simulink subsystem "subsistema_magnetico_estator"  (R2023b)
settings: Solver=VariableStepAuto  StartTime=0.0  StopTime=10.0  RelTol=1e-3
values from neighbouring files (symbols this model uses):
  L_d = 6.6    [main.m]    (also in parametros.m = 0.0066)
  L_q = 5.8e-3    (= 0.0058)    [diagrama_polos_y_ceros_LTI.m]    (also in main.m = 5.8; parametros.m; variacion_de_parametros.m)
  lambda_m = 0.016    [main.m]    (also in parametros.m)
  P_p = 3    [diagrama_polos_y_ceros_LTI.m]    (also in main.m; parametros.m; variacion_de_parametros.m)
settings Model: Creator=nicol  LastModifiedBy=nicol

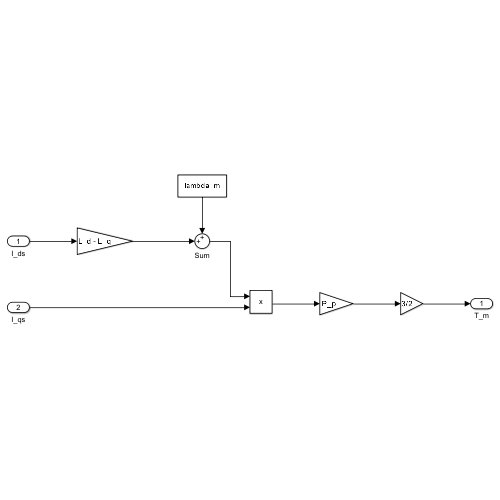
[thumbnail: Simulink's stored preview of the top-level diagram]
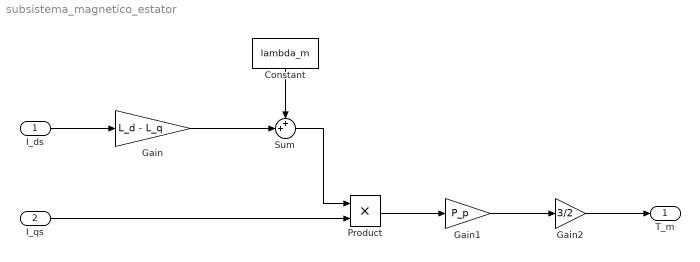
== system subsistema_magnetico_estator ==
  I_ds : Inport
  I_qs : Inport  Port=2
  Constant : Constant  Value=lambda_m
  Gain : Gain  Gain=L_d - L_q
  Gain1 : Gain  Gain=P_p
  Gain2 : Gain  Gain=3/2
  Product : Product
  Sum : Sum  Inputs=++|
  T_m : Outport
  wires:
  Sum/1 -> Product/1
  I_qs/1 -> Product/2
  Gain1/1 -> Gain2/1
  Product/1 -> Gain1/1
  Gain2/1 -> T_m/1
  Constant/1 -> Sum/1
  Gain/1 -> Sum/2
  I_ds/1 -> Gain/1
